simulink model "direct_form_II"  (R2015a)
settings: Solver=ode45  StartTime=0.0  StopTime=10.0  RelTol=1e-3
undefined symbols (not defined in the file): a1, a2, b0, b1, b2
settings Model: Creator=Lennon  LastModifiedBy=Lennon

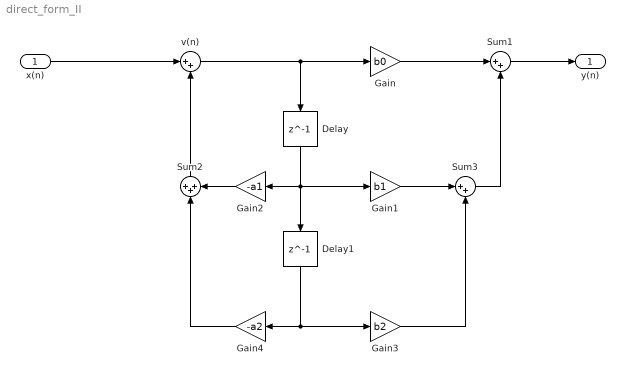
== system direct_form_II ==
  x(n) : Inport
  Delay : Delay  DelayLength=1  InitialCondition=0
  Delay1 : Delay  DelayLength=1  InitialCondition=0
  Gain : Gain  Gain=b0  ParamDataTypeStr=fixdt(1,16,2^0,0)  OutDataTypeStr=fixdt(1,16,2^0,0)  RndMeth=Round
  Gain1 : Gain  Gain=b1  ParamDataTypeStr=fixdt(1,16,2^0,0)  OutDataTypeStr=fixdt(1,16,2^0,0)  RndMeth=Round
  Gain2 : Gain  Gain=-a1  ParamDataTypeStr=fixdt(1,16,2^0,0)  OutDataTypeStr=fixdt(1,16,2^0,0)  RndMeth=Round
  Gain3 : Gain  Gain=b2  ParamDataTypeStr=fixdt(1,16,2^0,0)  OutDataTypeStr=fixdt(1,16,2^0,0)  RndMeth=Round
  Gain4 : Gain  Gain=-a2  ParamDataTypeStr=fixdt(1,16,2^0,0)  OutDataTypeStr=fixdt(1,16,2^0,0)  RndMeth=Round
  Sum1 : Sum  Inputs=|++  AccumDataTypeStr=fixdt(1,16,2^0,0)  OutDataTypeStr=fixdt(1,16,2^0,0)  RndMeth=Round
  Sum2 : Sum  Inputs=+++  AccumDataTypeStr=fixdt(1,16,2^0,0)  OutDataTypeStr=fixdt(1,16,2^0,0)  RndMeth=Round
  Sum3 : Sum  Inputs=|++  AccumDataTypeStr=fixdt(1,16,0)  OutDataTypeStr=fixdt(1,16,0)  RndMeth=Round
  "v(n) " : Sum  Inputs=|++  AccumDataTypeStr=fixdt(1,16,2^0,0)  OutDataTypeStr=fixdt(1,16,2^0,0)  RndMeth=Round
  y(n) : Outport
  wires:
  x(n)/1 -> "v(n) "/1
  "v(n) "/1 -> Delay/1, Gain/1
  Gain/1 -> Sum1/1
  Sum1/1 -> y(n)/1
  Delay1/1 -> Gain3/1, Gain4/1
  Delay/1 -> Gain2/1, Delay1/1, Gain1/1
  Gain4/1 -> Sum2/2
  Gain2/1 -> Sum2/3
  Sum2/1 -> "v(n) "/2
  Gain1/1 -> Sum3/1
  Sum3/1 -> Sum1/2
  Gain3/1 -> Sum3/2
